simulink model "main"  (R2021a)
settings: Solver=ode45  StartTime=0.0  StopTime=300  RelTol=1e-3
undefined symbols (not defined in the file or in its folder): Discrete, Earth, Time, WGS84
libraries: pid_lib x7, dspvision x5, simulink x2, dspindex x2, ctrlSharedLib x1, aerolibfltsims x1, aerolibtransform2 x1, dspsnks4 x1
(part 1 of 2)
settings Model: SimulationMode=accelerator  Creator=ZumoArthicha  LastModifiedBy=ZumoArthicha

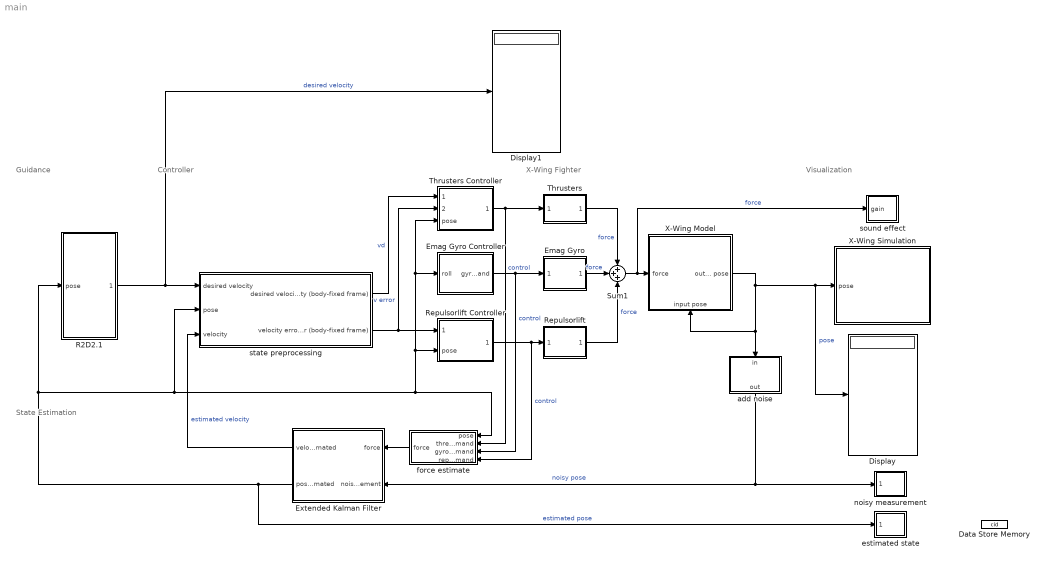
== system main ==
  note: Guidance
  note: Controller
  note: Visualization
  note: X-Wing Fighter
  note: State Estimation
  Data Store Memory : DataStoreMemory  DataStoreName=cid  ReadBeforeWriteMsg=warning  WriteAfterWriteMsg=warning  WriteAfterReadMsg=warning  ShowAdditionalParam=off
  Display : Display
  Display1 : Display
  Emag Gyro : Subsystem
      mask Display: image(imread("pictures/electromagneticgyro.PNG"))
  Emag Gyro Controller : Subsystem
      mask Display: image(imread("pictures/electromagneticgyro.PNG"))
  Extended Kalman Filter : Subsystem
      mask Display: image(imread("pictures/kalman.PNG"))
  R2D2.1 : Subsystem
      mask Display: image(imread("pictures/R2D2_crazy.PNG"))
  Repulsorlift : Subsystem
      mask Display: image(imread("pictures/repulserlift.PNG"))
  Repulsorlift Controller : Subsystem
      mask Display: image(imread("pictures/repulserlift.PNG"))
  Sum1 : Sum  Inputs=+++
  Thrusters : Subsystem
      mask Display: image(imread("pictures/thrusters.PNG"))
  Thrusters Controller : Subsystem
      mask Display: image(imread("pictures/thrusters.PNG"))
  X-Wing Model : Subsystem
      settings: PortSchema="{\"entries\":[{\"content\":{\"sides\":[{\"content\":{\"connectorIds\":[\"In1\"]},\"type\":\"ConnectorPlacement.EquallySpacedRectSide\",\"uuid\":\"9b8fdf7d-c3f6-4599-b802-210579db8a0c\"},{\"content\":{\"connectorIds\":[\"Out1\"],\"side\":\"RIGHT\"},\"type\":\"ConnectorPlacement.EquallySpacedRectSide\",\"uuid\":\"64fce1f1-7921-46e2-bebf-614926f0f3ad\"},{\"content\":{\"connectorIds\":[],\"side\":\"TOP\"},\"type\":\"ConnectorPlacement.EquallySpacedRectSide\",\"uuid\":\"e545f28f-71e6-4ea6-95f8-1eb7e380d19b\"},{\"content\":{\"connectorIds\":[\"In2\"],\"side\":\"BOTTOM\"},\"type\":\"ConnectorPlacement.EquallySpacedRectSide\",\"uuid\":\"bfd9a8ec-cd4d-4e0d-ab0a-253386349908\"}]},\"type\":\"ConnectorPlacement.EquallySpacedConnector\",\"uuid\":\"b40ebf44-1443-4f81-b67e-9daee8e56b53\"}],\"packageUris\":[\"http://schema.mathworks.com/mf0/Connector/R2020b\"],\"version\":\"1.0\"}"
      mask Display: image(imread("pictures/simplified_model.png"))
  X-Wing Simulation : Subsystem
      mask Display: image(imread("pictures/simulation.PNG"))
  add noise : Subsystem
      settings: PortSchema="{\"entries\":[{\"content\":{\"sides\":[{\"content\":{\"connectorIds\":[]},\"type\":\"ConnectorPlacement.EquallySpacedRectSide\",\"uuid\":\"f30e32c1-a276-4dc3-be84-096135bc4245\"},{\"content\":{\"connectorIds\":[],\"side\":\"RIGHT\"},\"type\":\"ConnectorPlacement.EquallySpacedRectSide\",\"uuid\":\"4791b214-a858-4f7a-9932-cf1e7f19f03d\"},{\"content\":{\"connectorIds\":[\"In1\"],\"side\":\"TOP\"},\"type\":\"ConnectorPlacement.EquallySpacedRectSide\",\"uuid\":\"5d6a58a2-1496-42ba-b7c9-fa854909925b\"},{\"content\":{\"connectorIds\":[\"Out1\"],\"side\":\"BOTTOM\"},\"type\":\"ConnectorPlacement.EquallySpacedRectSide\",\"uuid\":\"4cc45cbe-4744-429a-bad1-818b1ea51f93\"}]},\"type\":\"ConnectorPlacement.EquallySpacedConnector\",\"uuid\":\"9c6af004-83db-43a3-a1c2-cc96f6fd9fdc\"}],\"packageUris\":[\"http://schema.mathworks.com/mf0/Connector/R2020b\"],\"version\":\"1.0\"}"
      mask Display: image(imread("pictures/force.jpg"))
  estimated state : Subsystem
      mask Display: image(imread("pictures/xy_graph.png"))
  force estimate : Subsystem
      mask Display: image('D:\SDU\courses\F22_GuidanceNavigationAndControl\project\workspace\pictures\computer.jpg'); % Use "Edit Image" on toolstrip to change.
  noisy measurement : Subsystem
      mask Display: image(imread("pictures/xy_graph.png"))
  sound effect : Subsystem
      mask Display: image(imread("pictures/audio.PNG"))
  state preprocessing : Subsystem
  wires:
  X-Wing Model/1(output pose) -> X-Wing Model/2(input pose), add noise/1(in), Display/1, X-Wing Simulation/1(pose)  "pose"
  Thrusters Controller/1(thrusters command) -> Thrusters/1(threster command), force estimate/2(threster command)  "control"
  Repulsorlift Controller/1(repulsorlift command) -> force estimate/4(repulsorlift command), Repulsorlift/1(repulsorlift command)  "control"
  state preprocessing/1(desired velocity (body-fixed frame)) -> Thrusters Controller/1(desired velocity)  "vd"
  R2D2.1/1(desired velocity) -> Display1/1, state preprocessing/1(desired velocity)  "desired velocity"
  Emag Gyro Controller/1(gyros command) -> force estimate/3(gyros command), Emag Gyro/1(gyros command)  "control"
  Sum1/1 -> sound effect/1(gain), X-Wing Model/1(force)  "force"
  add noise/1(out) -> Extended Kalman Filter/2(noisy measurement), noisy measurement/1(" ")  "noisy pose"
  Extended Kalman Filter/2(pose estimated) -> R2D2.1/1(pose), state preprocessing/2(pose), force estimate/1(pose), Repulsorlift Controller/2(pose), Emag Gyro Controller/1(roll), Thrusters Controller/3(pose), estimated state/1(" ")  "estimated pose"
  Extended Kalman Filter/1(velocity estimated) -> state preprocessing/3(velocity)  "estimated velocity"
  Repulsorlift/1(repulsorlift force) -> Sum1/3  "force"
  Emag Gyro/1(gyros force) -> Sum1/2  "force"
  Thrusters/1(combined thrusters force) -> Sum1/1  "force"
  force estimate/1(force) -> Extended Kalman Filter/1(force)
  state preprocessing/2(velocity error (body-fixed frame)) -> Thrusters Controller/2(velocity error (body-fixed frame)), Repulsorlift Controller/1(vz error)  "v error"

== system main/Emag Gyro ==
  gyros command : Inport
  gyros force : Outport  PortDimensions=6
  wires:
  gyros command/1 -> gyros force/1

== system main/Emag Gyro Controller ==
  roll : Inport
  Constant : Constant  Value=0
  Demux5 : Demux  Outputs=6
  Gain : Gain  Gain=1e4
  Gyros PID : pid_lib/PID Controller  Controller=PID  Form=Parallel  TimeDomain=Continuous-time  UseExternalTs=off  SampleTime=-1  IntegratorMethod=Forward Euler  FilterMethod=Forward Euler  ControllerParametersSource=internal  P=0.5  I=0  D=1  UseFilter=on  N=100  TunerSelectOption=Transfer Function Based (PID Tuner App)  InitialConditionSource=internal  InitialConditionForIntegrator=0  InitialConditionForFilter=0  DifferentiatorICPrevScaledInput=0  ExternalReset=none  TrackingMode=off  Kt=1  LimitOutput=off  SatLimitsSource=internal  UpperSaturationLimit=inf  LowerSaturationLimit=-inf  LinearizeAsGain=on  AntiWindupMode=none  Kb=1  POutMin=[]  POutMax=[]  IOutMin=[]  IOutMax=[]  DOutMin=[]  DOutMax=[]  NOutMin=[]  NOutMax=[]  SumOutMin=[]  SumOutMax=[]  SaturationOutMin=[]  SaturationOutMax=[]  PParamMin=[]  PParamMax=[]  IParamMin=[]  IParamMax=[]  DParamMin=[]  DParamMax=[]  NParamMin=[]  NParamMax=[]  KbParamMin=[]  KbParamMax=[]  KtParamMin=[]  KtParamMax=[]  KbOutMin=[]  KbOutMax=[]  KtOutMin=[]  KtOutMax=[]  IntegratorOutMin=[]  IntegratorOutMax=[]  FilterOutMin=[]  FilterOutMax=[]  SumI1OutMin=[]  SumI1OutMax=[]  SumI2OutMin=[]  SumI2OutMax=[]  SumI3OutMin=[]  SumI3OutMax=[]  SumI4OutMin=[]  SumI4OutMax=[]  SumDOutMin=[]  SumDOutMax=[]  DifferentiatorOutMin=[]  DifferentiatorOutMax=[]  FilterDiffOutCoefMin=[]  FilterDiffOutCoefMax=[]  ReciprocalOutMin=[]  ReciprocalOutMax=[]  SumDenOutMin=[]  SumDenOutMax=[]  SumNumOutMin=[]  SumNumOutMax=[]  DivideOutMin=[]  DivideOutMax=[]  UdiffTsProdOutMin=[]  UdiffTsProdOutMax=[]  NTsProdOutMin=[]  NTsProdOutMax=[]  UintegralTsProdOutMin=[]  UintegralTsProdOutMax=[]  UngainTsProdOutMin=[]  UngainTsProdOutMax=[]  IntegratorContinuousStateAttributes=''  IntegratorStateMustResolveToSignalObject=off  IntegratorRTWStateStorageClass=Auto  FilterContinuousStateAttributes=''  FilterStateMustResolveToSignalObject=off  FilterRTWStateStorageClass=Auto  ParallelPVariant=InternalParameters  IdealPVariant=Disabled  IVariant=InternalParameters  DVariant=InternalParameters  IntegratorVariant=Continuous  SatVariant=Disabled  AWVariant=Passthrough  PCopyVariant=Disabled  TRVariant=Disabled  FdbkBlocksVariant=Forward  IdealPFdbkVariant=Disabled  SatFdbkVariant=Disabled  DerivativeFilterVariant=ContFilter  NVariant=InternalParameters  NCopyVariant=Disabled  FilterICVariant=InternalICsFilter  IntegratorICVariant=InternalICs  ExternalResetVariant=Disabled  TRSumVariant=Passthrough  SumFdbkVariant=Disabled  SumVariant=Sum_PID  TsampFilterVariant=InternalTs  TsampNgainVariant=Passthrough  TsampIntegralVariant=Passthrough  ExternalSaturationOutDataTypeStr=Inherit: Same as second input
  Product : Product
  Sum : Sum  Inputs=|+-
  directional constrain : Constant  Value=[0;0;0;1;0;0]  VectorParams1D=off
  gyros command : Outport  PortDimensions=6
  wires:
  directional constrain/1 -> Product/1  "directional constrain"
  Gain/1 -> Product/2
  Sum/1 -> Gyros PID/1  "roll error"
  Constant/1 -> Sum/1
  roll/1 -> Demux5/1
  Demux5/4 -> Sum/2
  Gyros PID/1 -> Gain/1
  Product/1 -> gyros command/1

== system main/Extended Kalman Filter ==
  force : Inport
  noisy measurement : Inport  Port=2
  Kalman Filter : Subsystem
      mask Display: image(imread("pictures/kalman.PNG"))
  To File : ToFile  Filename=pose.mat  MatrixName=data  SaveFormat=Timeseries
  input linearization : Subsystem
      mask Display: image(imread("pictures/equations/linearization.PNG"))
  velocity estimated : Outport
  pose estimated : Outport  Port=2
  wires:
  input linearization/1(force1) -> Kalman Filter/1(force)
  Kalman Filter/2(estimated velocity) -> velocity estimated/1  "velocity estimated"
  Kalman Filter/1(estimated pose) -> To File/1, input linearization/1(pose), pose estimated/1  "pose estimated"
  force/1 -> input linearization/2(force)
  noisy measurement/1 -> Kalman Filter/2(measure)

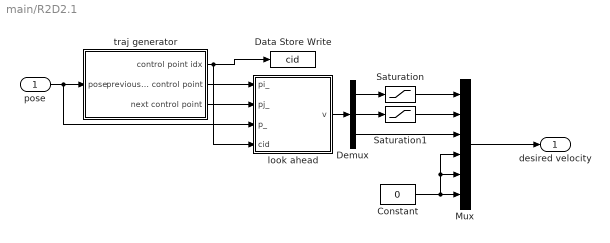
== system main/R2D2.1 ==
  pose : Inport
  Constant : Constant  Value=0
  Data Store Write : DataStoreWrite  DataStoreName=cid  IndexOptions=Index vector (dialog)  Indices=1  OutputSizes=1
  Demux : Demux  Outputs=3
  Mux : Mux  Inputs=6
  Saturation : Saturate  UpperLimit=100  LowerLimit=-100
  Saturation1 : Saturate  UpperLimit=100  LowerLimit=-100
  look ahead : MATLAB Function  TreatAsAtomicUnit=on
  traj generator : Subsystem
  desired velocity : Outport
  wires:
  traj generator/3(next control point) -> look ahead/2(pj_)
  pose/1 -> look ahead/3(p_), traj generator/1(pose)
  traj generator/2(previous control point) -> look ahead/1(pi_)
  look ahead/1(v) -> Demux/1
  Demux/3 -> Mux/3
  Constant/1 -> Mux/4, Mux/5, Mux/6
  Mux/1 -> desired velocity/1
  traj generator/1(control point idx) -> Data Store Write/1, look ahead/4(cid)
  Demux/2 -> Saturation1/1
  Demux/1 -> Saturation/1
  Saturation/1 -> Mux/1
  Saturation1/1 -> Mux/2

== system main/Repulsorlift ==
  repulsorlift command : Inport
  repulsorlift force : Outport  PortDimensions=6
  wires:
  repulsorlift command/1 -> repulsorlift force/1

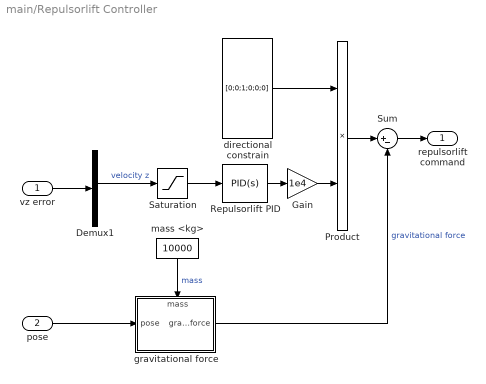
== system main/Repulsorlift Controller ==
  vz error : Inport
  pose : Inport  Port=2
  Demux1 : Demux  Outputs=6
  Gain : Gain  Gain=1e4
  Product : Product
  Repulsorlift PID : pid_lib/PID Controller  Controller=PID  Form=Parallel  TimeDomain=Continuous-time  UseExternalTs=off  SampleTime=-1  IntegratorMethod=Forward Euler  FilterMethod=Forward Euler  ControllerParametersSource=internal  P=0.01  I=0  D=0.1  UseFilter=on  N=100  TunerSelectOption=Transfer Function Based (PID Tuner App)  InitialConditionSource=internal  InitialConditionForIntegrator=0  InitialConditionForFilter=0  DifferentiatorICPrevScaledInput=0  ExternalReset=none  TrackingMode=off  Kt=1  LimitOutput=off  SatLimitsSource=internal  UpperSaturationLimit=inf  LowerSaturationLimit=-inf  LinearizeAsGain=on  AntiWindupMode=none  Kb=1  POutMin=[]  POutMax=[]  IOutMin=[]  IOutMax=[]  DOutMin=[]  DOutMax=[]  NOutMin=[]  NOutMax=[]  SumOutMin=[]  SumOutMax=[]  SaturationOutMin=[]  SaturationOutMax=[]  PParamMin=[]  PParamMax=[]  IParamMin=[]  IParamMax=[]  DParamMin=[]  DParamMax=[]  NParamMin=[]  NParamMax=[]  KbParamMin=[]  KbParamMax=[]  KtParamMin=[]  KtParamMax=[]  KbOutMin=[]  KbOutMax=[]  KtOutMin=[]  KtOutMax=[]  IntegratorOutMin=[]  IntegratorOutMax=[]  FilterOutMin=[]  FilterOutMax=[]  SumI1OutMin=[]  SumI1OutMax=[]  SumI2OutMin=[]  SumI2OutMax=[]  SumI3OutMin=[]  SumI3OutMax=[]  SumI4OutMin=[]  SumI4OutMax=[]  SumDOutMin=[]  SumDOutMax=[]  DifferentiatorOutMin=[]  DifferentiatorOutMax=[]  FilterDiffOutCoefMin=[]  FilterDiffOutCoefMax=[]  ReciprocalOutMin=[]  ReciprocalOutMax=[]  SumDenOutMin=[]  SumDenOutMax=[]  SumNumOutMin=[]  SumNumOutMax=[]  DivideOutMin=[]  DivideOutMax=[]  UdiffTsProdOutMin=[]  UdiffTsProdOutMax=[]  NTsProdOutMin=[]  NTsProdOutMax=[]  UintegralTsProdOutMin=[]  UintegralTsProdOutMax=[]  UngainTsProdOutMin=[]  UngainTsProdOutMax=[]  IntegratorContinuousStateAttributes=''  IntegratorStateMustResolveToSignalObject=off  IntegratorRTWStateStorageClass=Auto  FilterContinuousStateAttributes=''  FilterStateMustResolveToSignalObject=off  FilterRTWStateStorageClass=Auto  ParallelPVariant=InternalParameters  IdealPVariant=Disabled  IVariant=InternalParameters  DVariant=InternalParameters  IntegratorVariant=Continuous  SatVariant=Disabled  AWVariant=Passthrough  PCopyVariant=Disabled  TRVariant=Disabled  FdbkBlocksVariant=Forward  IdealPFdbkVariant=Disabled  SatFdbkVariant=Disabled  DerivativeFilterVariant=ContFilter  NVariant=InternalParameters  NCopyVariant=Disabled  FilterICVariant=InternalICsFilter  IntegratorICVariant=InternalICs  ExternalResetVariant=Disabled  TRSumVariant=Passthrough  SumFdbkVariant=Disabled  SumVariant=Sum_PID  TsampFilterVariant=InternalTs  TsampNgainVariant=Passthrough  TsampIntegralVariant=Passthrough  ExternalSaturationOutDataTypeStr=Inherit: Same as second input
  Saturation : Saturate  UpperLimit=10  LowerLimit=-10
  Sum : Sum  Inputs=|+-
  directional constrain : Constant  Value=[0;0;1;0;0;0]  VectorParams1D=off
  gravitational force : Subsystem
      settings: PortSchema="{\"entries\":[{\"content\":{\"sides\":[{\"content\":{\"connectorIds\":[\"In1\"]},\"type\":\"ConnectorPlacement.EquallySpacedRectSide\",\"uuid\":\"d93db66b-fcc6-4c17-9134-40d9beba2643\"},{\"content\":{\"connectorIds\":[\"Out1\"],\"side\":\"RIGHT\"},\"type\":\"ConnectorPlacement.EquallySpacedRectSide\",\"uuid\":\"70571ecc-e0da-42b3-8b7b-d4ce677f32d8\"},{\"content\":{\"connectorIds\":[\"In2\"],\"side\":\"TOP\"},\"type\":\"ConnectorPlacement.EquallySpacedRectSide\",\"uuid\":\"56b2d7be-0ac4-47dc-afb8-3ce057fd0ced\"},{\"content\":{\"connectorIds\":[],\"side\":\"BOTTOM\"},\"type\":\"ConnectorPlacement.EquallySpacedRectSide\",\"uuid\":\"175b75d5-a12f-4632-9256-2a0db7457e72\"}]},\"type\":\"ConnectorPlacement.EquallySpacedConnector\",\"uuid\":\"6f54763d-dba9-4fd6-aa24-fb7b6af2d4a1\"}],\"packageUris\":[\"http://schema.mathworks.com/mf0/Connector/R2020b\"],\"version\":\"1.0\"}"
      mask Display: image(imread("pictures/gravitational_force.PNG"))
  mass <kg> : Constant  Value=10000
  repulsorlift command : Outport  PortDimensions=6
  wires:
  directional constrain/1 -> Product/1
  Repulsorlift PID/1 -> Gain/1
  Product/1 -> Sum/1
  Sum/1 -> repulsorlift command/1
  Gain/1 -> Product/2
  Saturation/1 -> Repulsorlift PID/1
  vz error/1 -> Demux1/1
  Demux1/3 -> Saturation/1  "velocity z"
  mass <kg>/1 -> gravitational force/2(mass)  "mass"
  pose/1 -> gravitational force/1(pose)
  gravitational force/1(gravitational force) -> Sum/2  "gravitational force"

== system main/Thrusters ==
  threster command : Inport  PortDimensions=4
  Matrix Multiply2 : Product  Multiplication=Matrix(*)
  thrust matrix : Constant  Value=[0.25 0.25 0.25 0.25; 0 0 0 0; 0 0 0 0; 0 0 0 0; -0.68 -0.68 0.68 0.68; 1.425 -1.425 1.425 -1.425]  VectorParams1D=off
  combined thrusters force : Outport  PortDimensions=6
  wires:
  thrust matrix/1 -> Matrix Multiply2/1
  Matrix Multiply2/1 -> combined thrusters force/1  "low-level thruster command"
  threster command/1 -> Matrix Multiply2/2

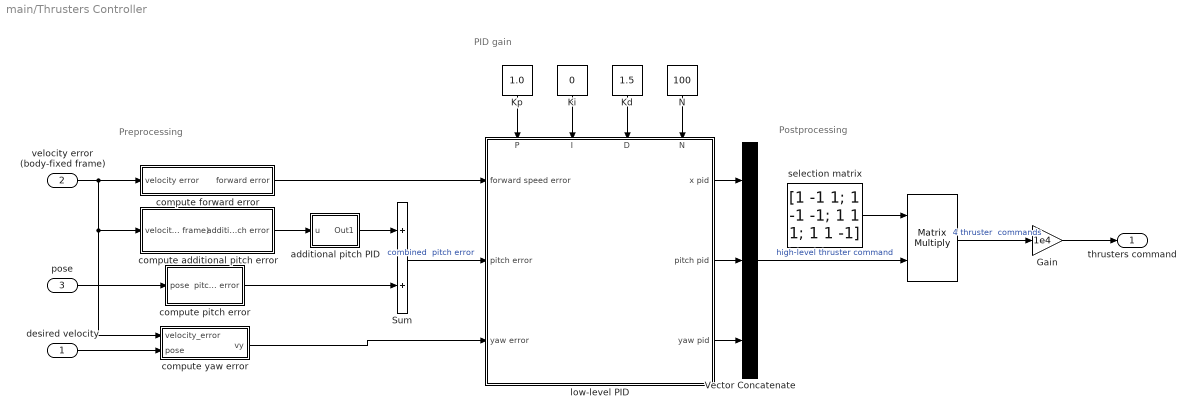
== system main/Thrusters Controller ==
  note: Postprocessing
  note: Preprocessing
  note: PID gain
  desired velocity : Inport
  velocity error (body-fixed frame) : Inport  Port=2
  pose : Inport  Port=3
  "  " : Product  Multiplication=Matrix(*)
  Gain : Gain  Gain=1e4
  Kd : Constant  Value=1.5
  Ki : Constant  Value=0
  Kp : Constant  Value=1.0
  N : Constant  Value=100
  Sum : Sum
  Vector Concatenate : Concatenate  NumInputs=3
  additional pitch PID : Subsystem
  compute additional pitch error : Subsystem
  compute forward error : Subsystem
  compute pitch error : Subsystem
  compute yaw error : Subsystem
  low-level PID : Subsystem
      settings: PortSchema="{\"entries\":[{\"content\":{\"sides\":[{\"content\":{\"connectorIds\":[\"In1\",\"In2\",\"In3\"]},\"type\":\"ConnectorPlacement.EquallySpacedRectSide\",\"uuid\":\"f6ea6f6d-4efd-425d-8a85-ce3b9bde565c\"},{\"content\":{\"connectorIds\":[\"Out1\",\"Out2\",\"Out3\"],\"side\":\"RIGHT\"},\"type\":\"ConnectorPlacement.EquallySpacedRectSide\",\"uuid\":\"bea2efba-fcca-41fe-8e46-9fa204d644b4\"},{\"content\":{\"connectorIds\":[\"In4\",\"In5\",\"In6\",\"In7\"],\"side\":\"TOP\"},\"type\":\"ConnectorPlacement.EquallySpacedRectSide\",\"uuid\":\"c7db24d1-2300-4d89-a06d-38d8ccf635f0\"}]},\"type\":\"ConnectorPlacement.EquallySpacedConnector\",\"uuid\":\"54c313d2-af5a-49ea-a2f4-4d36f80b668a\"}],\"packageUris\":[\"http://schema.mathworks.com/mf0/Connector/R2020b\"],\"version\":\"1.0\"}"
  selection matrix : Constant  Value=[1 -1 1; 1 -1 -1; 1 1 1; 1 1 -1]  VectorParams1D=off
  thrusters command : Outport  PortDimensions=4
  wires:
  Kp/1 -> low-level PID/4(P)
  selection matrix/1 -> "  "/1
  Vector Concatenate/1 -> "  "/2  "high-level thruster command"
  pose/1 -> compute pitch error/1(pose)
  compute pitch error/1(pitch error) -> Sum/2
  velocity error (body-fixed frame)/1 -> compute yaw error/1(velocity_error), compute additional pitch error/1(velocity error (world-fixed frame)), compute forward error/1(velocity error)
  desired velocity/1 -> compute yaw error/2(pose)
  compute additional pitch error/1(addition pitch error) -> additional pitch PID/1(u)
  additional pitch PID/1(Out1) -> Sum/1
  Ki/1 -> low-level PID/5(I)
  Kd/1 -> low-level PID/6(D)
  N/1 -> low-level PID/7(N)
  compute forward error/1(forward error) -> low-level PID/1(forward speed error)
  Sum/1 -> low-level PID/2(pitch error)  "combined  pitch error"
  compute yaw error/1(vy) -> low-level PID/3(yaw error)
  low-level PID/1(x pid) -> Vector Concatenate/1
  low-level PID/2(pitch pid) -> Vector Concatenate/2
  low-level PID/3(yaw pid) -> Vector Concatenate/3
  "  "/1 -> Gain/1  "4 thruster  commands"
  Gain/1 -> thrusters command/1

== system main/X-Wing Model ==
  force : Inport
  input pose : Inport  Port=2
  Sum : Sum  Inputs=++|
  X-wing Model : Subsystem
      settings: PortSchema="{\"entries\":[{\"content\":{\"sides\":[{\"content\":{\"connectorIds\":[\"In1\"]},\"type\":\"ConnectorPlacement.EquallySpacedRectSide\",\"uuid\":\"7004d7e2-eb30-41ed-9d5e-f00159415fc4\"},{\"content\":{\"connectorIds\":[\"Out1\",\"Out2\"],\"side\":\"RIGHT\"},\"type\":\"ConnectorPlacement.EquallySpacedRectSide\",\"uuid\":\"4cf7ba01-0c86-439c-9faf-473746ab50fc\"},{\"content\":{\"connectorIds\":[\"In2\",\"In3\"],\"side\":\"TOP\"},\"type\":\"ConnectorPlacement.EquallySpacedRectSide\",\"uuid\":\"4a15a873-16d7-4740-9282-1fecb26c48e4\"},{\"content\":{\"connectorIds\":[],\"side\":\"BOTTOM\"},\"type\":\"ConnectorPlacement.EquallySpacedRectSide\",\"uuid\":\"87e73f3e-eb46-42cc-8158-d40318a5aa75\"}]},\"type\":\"ConnectorPlacement.EquallySpacedConnector\",\"uuid\":\"64dad74e-3dd4-4677-9bab-84aaaaaa8f26\"}],\"packageUris\":[\"http://schema.mathworks.com/mf0/Connector/R2020b\"],\"version\":\"1.0\"}"
      mask Display: image(imread("pictures/simplified_model.png"))
  gravitational force : Subsystem
      settings: PortSchema="{\"entries\":[{\"content\":{\"sides\":[{\"content\":{\"connectorIds\":[\"In1\"]},\"type\":\"ConnectorPlacement.EquallySpacedRectSide\",\"uuid\":\"d93db66b-fcc6-4c17-9134-40d9beba2643\"},{\"content\":{\"connectorIds\":[\"Out1\"],\"side\":\"RIGHT\"},\"type\":\"ConnectorPlacement.EquallySpacedRectSide\",\"uuid\":\"70571ecc-e0da-42b3-8b7b-d4ce677f32d8\"},{\"content\":{\"connectorIds\":[\"In2\"],\"side\":\"TOP\"},\"type\":\"ConnectorPlacement.EquallySpacedRectSide\",\"uuid\":\"56b2d7be-0ac4-47dc-afb8-3ce057fd0ced\"},{\"content\":{\"connectorIds\":[],\"side\":\"BOTTOM\"},\"type\":\"ConnectorPlacement.EquallySpacedRectSide\",\"uuid\":\"175b75d5-a12f-4632-9256-2a0db7457e72\"}]},\"type\":\"ConnectorPlacement.EquallySpacedConnector\",\"uuid\":\"6f54763d-dba9-4fd6-aa24-fb7b6af2d4a1\"}],\"packageUris\":[\"http://schema.mathworks.com/mf0/Connector/R2020b\"],\"version\":\"1.0\"}"
      mask Display: image(imread("pictures/gravitational_force.PNG"))
  innertia <kg m2> : Constant  Value=[36145 0 0; 2.26927 116437.915354 0.00035374516; 0 0.00035374516 90590.2796914]  VectorParams1D=off
  mass <kg> : Constant  Value=10000
  output pose : Outport
  wires:
  mass <kg>/1 -> gravitational force/2(mass), X-wing Model/2(mass)  "mass"
  innertia <kg m2>/1 -> X-wing Model/3(inertia)  "inertia"
  X-wing Model/1(pose) -> output pose/1  "pose"
  input pose/1 -> gravitational force/1(pose)  "pose"
  Sum/1 -> X-wing Model/1(force)  "force"
  force/1 -> Sum/1
  gravitational force/1(gravitational force) -> Sum/2  "gravitational force"

== system main/X-Wing Simulation ==
  pose : Inport
  Constant1 : Constant  Value=[30;300;100]  VectorParams1D=off
  Demux : Demux  Outputs=2
  FlightGear Simulation : aerolibfltsims/FlightGear Preconfigured 6DoF Animation  xFlightGearVersion=v2019.1  DestinationIpAddress=127.0.0.1  DestinationPort=5502  SampleTime=1/20  packetVersion=24  mask(FlightGearQuick6DoFAnimation){}
      mask Display:
      | % This is a new mask on top of the base mask.
      | % Use "View base mask" link below to see the base mask.
      | image(imread("pictures/simulation.PNG"))
  MATLAB Function : MATLAB Function  TreatAsAtomicUnit=on
  Mux1 : Mux  Inputs=2
  flat earth 2 LLA : Subsystem
  special : Subsystem
  wires:
  MATLAB Function/1(pose_) -> FlightGear Simulation/1
  pose/1 -> Demux/1
  Demux/2 -> Mux1/2
  Mux1/1 -> MATLAB Function/1(pose)
  Constant1/1 -> flat earth 2 LLA/1(multiplication gain)
  Demux/1 -> flat earth 2 LLA/2(position (flat))
  flat earth 2 LLA/1(position (LLA)) -> Mux1/1

== system main/add noise ==
  in : Inport
  Measurement Noise : Subsystem
  Sum : Sum  Inputs=|++
  To File1 : ToFile  Filename=noisypose.mat  MatrixName=data  SaveFormat=Timeseries
  To File3 : ToFile  Filename=truepose.mat  MatrixName=data  SaveFormat=Timeseries
  out : Outport
  wires:
  Measurement Noise/1(nois) -> Sum/2
  in/1 -> To File3/1, Sum/1
  Sum/1 -> To File1/1, out/1  "measurement"

== system main/estimated state ==
  " " : Inport
  Demux3 : Demux  Outputs=6
  XY Graph : simulink/Sinks/XY Graph  xmin=-0.2  xmax=1  ymin=-0.2  ymax=1  st=-1
  scaling gain : Gain  Gain=2e-4
  wires:
  Demux3/1 -> XY Graph/1  "x"
  Demux3/2 -> XY Graph/2  "y"
  scaling gain/1 -> Demux3/1
  " "/1 -> scaling gain/1

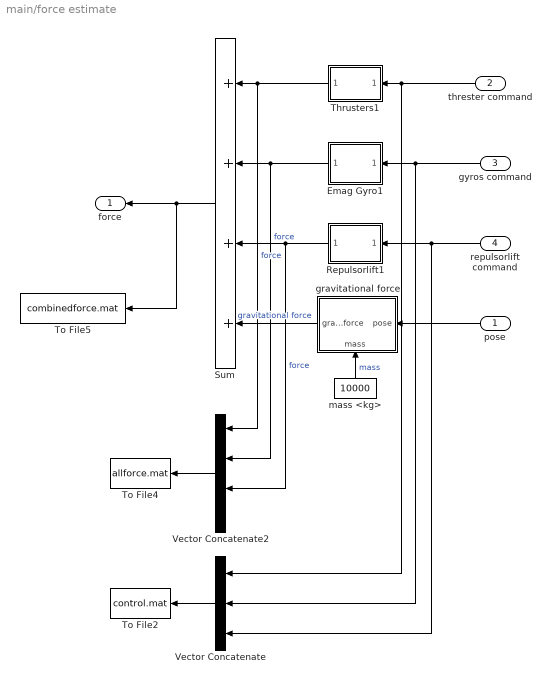
== system main/force estimate ==
  pose : Inport
  threster command : Inport  Port=2
  gyros command : Inport  Port=3
  repulsorlift command : Inport  Port=4
  Emag Gyro1 : Subsystem
      mask Display: image(imread("pictures/electromagneticgyro.PNG"))
  Repulsorlift1 : Subsystem
      mask Display: image(imread("pictures/repulserlift.PNG"))
  Sum : Sum  Inputs=++++
  Thrusters1 : Subsystem
      mask Display: image(imread("pictures/thrusters.PNG"))
  To File2 : ToFile  Filename=control.mat  MatrixName=data  SaveFormat=Timeseries
  To File4 : ToFile  Filename=allforce.mat  MatrixName=data  SaveFormat=Timeseries
  To File5 : ToFile  Filename=combinedforce.mat  MatrixName=data  SaveFormat=Timeseries
  Vector Concatenate : Concatenate  NumInputs=3
  Vector Concatenate2 : Concatenate  NumInputs=4
  gravitational force : Subsystem
      settings: PortSchema="{\"entries\":[{\"content\":{\"sides\":[{\"content\":{\"connectorIds\":[\"In1\"]},\"type\":\"ConnectorPlacement.EquallySpacedRectSide\",\"uuid\":\"d93db66b-fcc6-4c17-9134-40d9beba2643\"},{\"content\":{\"connectorIds\":[\"Out1\"],\"side\":\"RIGHT\"},\"type\":\"ConnectorPlacement.EquallySpacedRectSide\",\"uuid\":\"70571ecc-e0da-42b3-8b7b-d4ce677f32d8\"},{\"content\":{\"connectorIds\":[],\"side\":\"TOP\"},\"type\":\"ConnectorPlacement.EquallySpacedRectSide\",\"uuid\":\"56b2d7be-0ac4-47dc-afb8-3ce057fd0ced\"},{\"content\":{\"connectorIds\":[\"In2\"],\"side\":\"BOTTOM\"},\"type\":\"ConnectorPlacement.EquallySpacedRectSide\",\"uuid\":\"175b75d5-a12f-4632-9256-2a0db7457e72\"}]},\"type\":\"ConnectorPlacement.EquallySpacedConnector\",\"uuid\":\"6f54763d-dba9-4fd6-aa24-fb7b6af2d4a1\"}],\"packageUris\":[\"http://schema.mathworks.com/mf0/Connector/R2020b\"],\"version\":\"1.0\"}"
      mask Display: image(imread("pictures/gravitational_force.PNG"))
  mass <kg> : Constant  Value=10000
  force : Outport
  wires:
  gyros command/1 -> Vector Concatenate/2, Emag Gyro1/1(gyros command)
  threster command/1 -> Vector Concatenate/1, Thrusters1/1(threster command)
  repulsorlift command/1 -> Vector Concatenate/3, Repulsorlift1/1(repulsorlift command)
  Sum/1 -> To File5/1, force/1
  Emag Gyro1/1(gyros force) -> Vector Concatenate2/2, Sum/2  "force"
  Thrusters1/1(combined thrusters force) -> Vector Concatenate2/1, Sum/1  "force"
  Repulsorlift1/1(repulsorlift force) -> Vector Concatenate2/3, Sum/3  "force"
  Vector Concatenate2/1 -> To File4/1
  Vector Concatenate/1 -> To File2/1
  gravitational force/1(gravitational force) -> Sum/4  "gravitational force"
  pose/1 -> gravitational force/1(pose)
  mass <kg>/1 -> gravitational force/2(mass)  "mass"

== system main/noisy measurement ==
  " " : Inport
  Demux3 : Demux  Outputs=6
  XY Graph : simulink/Sinks/XY Graph  xmin=-0.2  xmax=1  ymin=-0.2  ymax=1  st=-1
  scaling gain : Gain  Gain=2e-4
  wires:
  Demux3/1 -> XY Graph/1  "x"
  Demux3/2 -> XY Graph/2  "y"
  scaling gain/1 -> Demux3/1
  " "/1 -> scaling gain/1

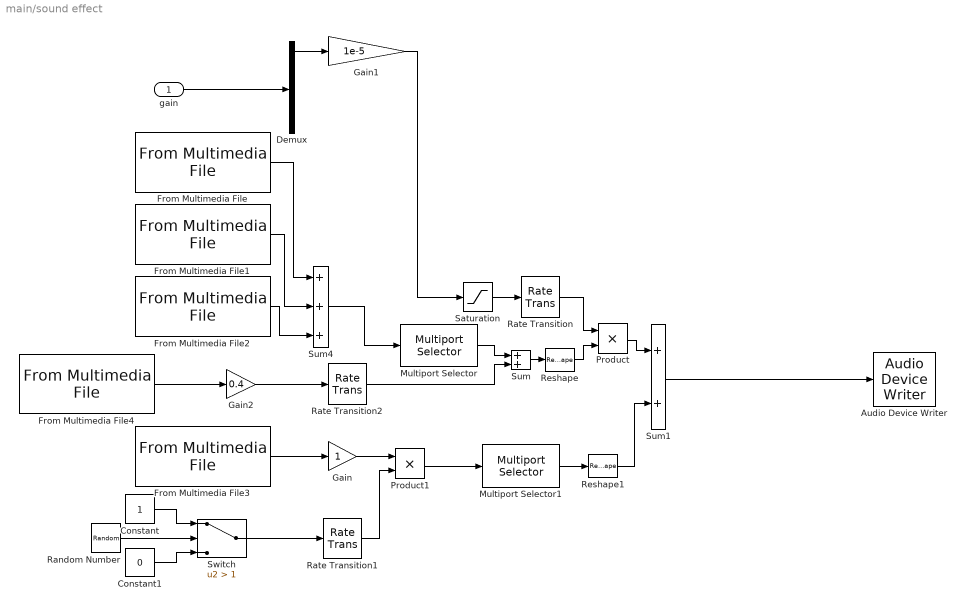
== system main/sound effect ==
  gain : Inport
  Audio Device Writer : dspsnks4/Audio Device Writer  Driver=DirectSound  Device=Default  InheritSampleRate=on  SampleRate=44100  BitDepth=16-bit integer  BufferSize=4096  NumBuffers=10  DefaultOutputChannelMapping=on  OutputChannelMapping=1:2  OutputNumUnderrunSamples=off  DriverIdx=1  DeviceWarnFlag=''
  Constant : Constant
  Constant1 : Constant  Value=0
  Demux : Demux  Outputs=6
  From Multimedia File : dspvision/From Multimedia File  inputFilename=D:\SDU\courses\F22_GuidanceNavigationAndControl\project\workspace\sound\XWing-Fly1.wav  readRange=[1 Inf]  loop=on  numPlays=inf  outputStreams=Audio only  videoDataType=single  audioDataType=double  inheritSampleTime=on  userDefinedSampleTime=1/30  noAudioOutput=off  isIntensityVideo=off  fourcc=RGB  colorVideoFormat=One multidimensional signal  outputEOF=off  dataOrg=Column-major  audioFrameSize=1024  computeAudioFrameSize=off  outSamplingMode=Sample based
  From Multimedia File1 : dspvision/From Multimedia File  inputFilename=D:\SDU\courses\F22_GuidanceNavigationAndControl\project\workspace\sound\XWing-Fly2.wav  readRange=[1 Inf]  loop=on  numPlays=inf  outputStreams=Audio only  videoDataType=single  audioDataType=double  inheritSampleTime=on  userDefinedSampleTime=1/30  noAudioOutput=off  isIntensityVideo=off  fourcc=RGB  colorVideoFormat=One multidimensional signal  outputEOF=off  dataOrg=Column-major  audioFrameSize=1024  computeAudioFrameSize=off  outSamplingMode=Sample based
  From Multimedia File2 : dspvision/From Multimedia File  inputFilename=D:\SDU\courses\F22_GuidanceNavigationAndControl\project\workspace\sound\XWing-Fly3.wav  readRange=[1 Inf]  loop=on  numPlays=inf  outputStreams=Audio only  videoDataType=single  audioDataType=double  inheritSampleTime=on  userDefinedSampleTime=1/30  noAudioOutput=off  isIntensityVideo=off  fourcc=RGB  colorVideoFormat=One multidimensional signal  outputEOF=off  dataOrg=Column-major  audioFrameSize=1024  computeAudioFrameSize=off  outSamplingMode=Sample based
  From Multimedia File3 : dspvision/From Multimedia File  inputFilename=D:\SDU\courses\F22_GuidanceNavigationAndControl\project\workspace\sound\XWing-Laser.wav  readRange=[1 Inf]  loop=on  numPlays=inf  outputStreams=Audio only  videoDataType=single  audioDataType=double  inheritSampleTime=on  userDefinedSampleTime=1/30  noAudioOutput=off  isIntensityVideo=off  fourcc=RGB  colorVideoFormat=One multidimensional signal  outputEOF=off  dataOrg=Column-major  audioFrameSize=1024  computeAudioFrameSize=off  outSamplingMode=Sample based
  From Multimedia File4 : dspvision/From Multimedia File  inputFilename=D:\SDU\courses\F22_GuidanceNavigationAndControl\project\workspace\sound\R2D2.mp3  readRange=[1 Inf]  loop=on  numPlays=inf  outputStreams=Audio only  videoDataType=single  audioDataType=double  inheritSampleTime=on  userDefinedSampleTime=1/30  noAudioOutput=off  isIntensityVideo=off  fourcc=RGB  colorVideoFormat=One multidimensional signal  outputEOF=off  dataOrg=Column-major  audioFrameSize=1024  computeAudioFrameSize=off  outSamplingMode=Sample based
  Gain : Gain
  Gain1 : Gain  Gain=1e-5
  Gain2 : Gain  Gain=0.4
  Multiport Selector : dspindex/Multiport Selector  rowsOrCols=Columns  idxCellArray=2  idxErrMode=Clip Index
  Multiport Selector1 : dspindex/Multiport Selector  rowsOrCols=Columns  idxCellArray=2  idxErrMode=Clip Index
  Product : Product
  Product1 : Product
  Random Number : RandomNumber  SampleTime=0.4643990929705216
  Rate Transition : RateTransition
  Rate Transition1 : RateTransition
  Rate Transition2 : RateTransition
  Reshape : Reshape
  Reshape1 : Reshape
  Saturation : Saturate  UpperLimit=1  LowerLimit=0.5
  Sum : Sum
  Sum1 : Sum
  Sum4 : Sum  Inputs=+++
  Switch : Switch  Criteria=u2 > Threshold  Threshold=1
  wires:
  From Multimedia File3/1 -> Gain/1
  From Multimedia File/1 -> Sum4/1
  From Multimedia File2/1 -> Sum4/3
  From Multimedia File1/1 -> Sum4/2
  Product/1 -> Sum1/1
  Sum1/1 -> Audio Device Writer/1
  Sum4/1 -> Multiport Selector/1
  Multiport Selector1/1 -> Reshape1/1
  Demux/1 -> Gain1/1
  gain/1 -> Demux/1
  Gain1/1 -> Saturation/1
  Rate Transition/1 -> Product/1
  Reshape1/1 -> Sum1/2
  Saturation/1 -> Rate Transition/1
  Gain/1 -> Product1/1
  Product1/1 -> Multiport Selector1/1
  Rate Transition1/1 -> Product1/2
  Random Number/1 -> Switch/2
  Constant/1 -> Switch/1
  Constant1/1 -> Switch/3
  Switch/1 -> Rate Transition1/1
  From Multimedia File4/1 -> Gain2/1
  Reshape/1 -> Product/2
  Sum/1 -> Reshape/1
  Multiport Selector/1 -> Sum/1
  Rate Transition2/1 -> Sum/2
  Gain2/1 -> Rate Transition2/1

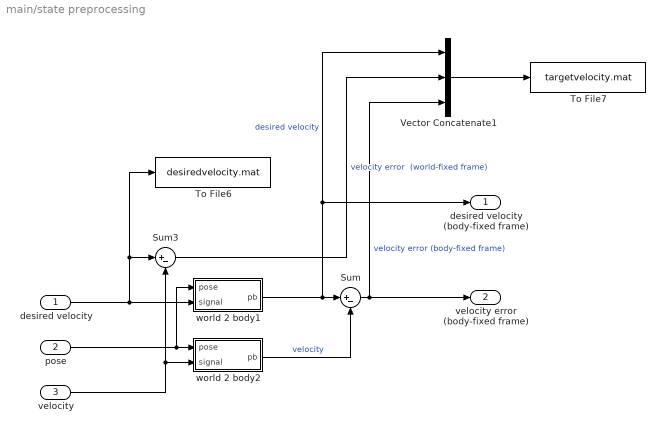
== system main/state preprocessing ==
  desired velocity : Inport
  pose : Inport  Port=2
  velocity : Inport  Port=3
  Sum : Sum  Inputs=|+-
  Sum3 : Sum  Inputs=|+-
  To File6 : ToFile  Filename=desiredvelocity.mat  MatrixName=data  SaveFormat=Timeseries
  To File7 : ToFile  Filename=targetvelocity.mat  MatrixName=data  SaveFormat=Timeseries
  Vector Concatenate1 : Concatenate  NumInputs=3
  world 2 body1 : MATLAB Function  TreatAsAtomicUnit=on
  world 2 body2 : MATLAB Function  TreatAsAtomicUnit=on
  desired velocity (body-fixed frame) : Outport
  velocity error (body-fixed frame) : Outport  Port=2
  wires:
  world 2 body1/1(pb) -> Vector Concatenate1/1, desired velocity (body-fixed frame)/1, Sum/1  "desired velocity"
  desired velocity/1 -> world 2 body1/2(signal), To File6/1, Sum3/1
  Sum/1 -> Vector Concatenate1/3, velocity error (body-fixed frame)/1  "velocity error (body-fixed frame)"
  pose/1 -> world 2 body1/1(pose), world 2 body2/1(pose)
  world 2 body2/1(pb) -> Sum/2  "velocity"
  Sum3/1 -> Vector Concatenate1/2  "velocity error  (world-fixed frame)"
  velocity/1 -> world 2 body2/2(signal), Sum3/2
  Vector Concatenate1/1 -> To File7/1

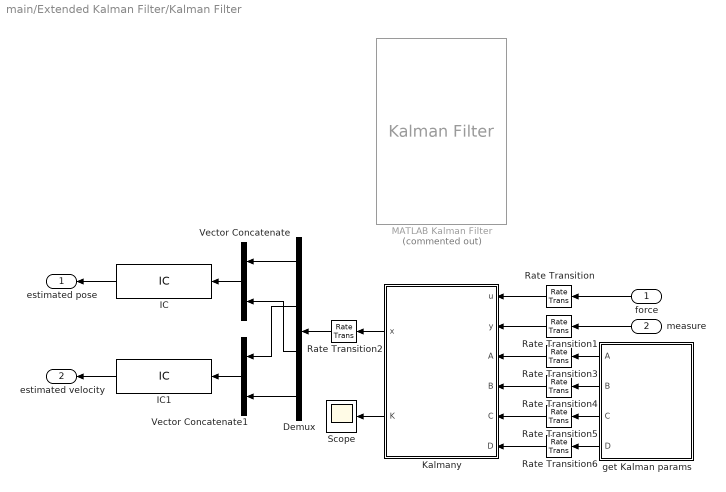
== system main/Extended Kalman Filter/Kalman Filter ==
  force : Inport
  measure : Inport  Port=2
  Demux : Demux
  IC : InitialCondition  Value=[0;0;1.705/100;0;0;0]
  IC1 : InitialCondition  Value=[0;0;0;0;0;0]
  Kalmany : Subsystem
  MATLAB Kalman Filter : ctrlSharedLib/Kalman Filter  Commented=on  TimeDomain=Discrete-Time  UseCurrentEstimator=on  ModelSource=Input port  ModelSourceVariable=ss(0.95,1,1,0,1)  A=0.95  B=1  C=1  D=0  NumberOfStates=12  NumberOfInputs=6  NumberOfOutputs=6  InitialEstimateSource=Dialog  X0=[0;0;1.705/100;0;0;0;0;0;0;0;0;0]  P0=10  UseK=off  UseGH=off  NumberOfProcessNoiseInputs=1  G=1  TimeInvariantG=on  H=0  TimeInvariantH=on  Q=1  TimeInvariantQ=on  R=100  TimeInvariantR=on  N=0  TimeInvariantN=on  AddInputPort=on  AddEnablePort=off  OutputEstimatedY=off  OutputP=off  Ts=0.005
  Rate Transition{,1,3..6} (6 alike) : RateTransition  OutPortSampleTime=0.005
  Rate Transition2 : RateTransition  OutPortSampleTime=0
  Scope : Scope
  Vector Concatenate : Concatenate
  Vector Concatenate1 : Concatenate
  get Kalman params : MATLAB Function  TreatAsAtomicUnit=on
  estimated pose : Outport
  estimated velocity : Outport  Port=2
  wires:
  force/1 -> Rate Transition/1
  measure/1 -> Rate Transition1/1
  Vector Concatenate1/1 -> IC1/1
  Demux/2 -> Vector Concatenate1/1
  Demux/1 -> Vector Concatenate/1
  Demux/3 -> Vector Concatenate/2
  Vector Concatenate/1 -> IC/1
  Demux/4 -> Vector Concatenate1/2
  Rate Transition2/1 -> Demux/1
  IC/1 -> estimated pose/1
  IC1/1 -> estimated velocity/1
  get Kalman params/1(A) -> Rate Transition3/1
  get Kalman params/2(B) -> Rate Transition4/1
  get Kalman params/4(D) -> Rate Transition6/1
  get Kalman params/3(C) -> Rate Transition5/1
  Rate Transition/1 -> Kalmany/1(u)
  Rate Transition1/1 -> Kalmany/2(y)
  Rate Transition3/1 -> Kalmany/3(A)
  Rate Transition4/1 -> Kalmany/4(B)
  Rate Transition5/1 -> Kalmany/5(C)
  Rate Transition6/1 -> Kalmany/6(D)
  Kalmany/1(x) -> Rate Transition2/1
  Kalmany/2(K) -> Scope/1

== system main/Extended Kalman Filter/input linearization ==
  pose : Inport
  force : Inport  Port=2
  body 2 world 1 : MATLAB Function  TreatAsAtomicUnit=on
  force1 : Outport
  wires:
  pose/1 -> body 2 world 1/2(pose)
  body 2 world 1/1(pb) -> force1/1  "force"
  force/1 -> body 2 world 1/1(signal)

== system main/R2D2.1/traj generator ==
  pose : Inport
  Integrator : Integrator  InitialCondition=2
  trajectory gens : MATLAB Function  TreatAsAtomicUnit=on
  control point idx : Outport  PortDimensions=1
  previous control point : Outport  Port=2  PortDimensions=3
  next control point : Outport  Port=3  PortDimensions=3
  wires:
  trajectory gens/1(posei) -> previous control point/1
  pose/1 -> trajectory gens/1(fb)
  trajectory gens/3(added_idx) -> Integrator/1
  Integrator/1 -> control point idx/1, trajectory gens/2(idx)
  trajectory gens/2(posej) -> next control point/1

== system main/Repulsorlift Controller/gravitational force ==
  pose : Inport
  mass : Inport  Port=2
  Subsystem : Subsystem
      mask Display: image(imread("pictures/equations/gravitational_force.png"))
  gravitational force visualization : Scope  Commented=on
  "world 2 body " : MATLAB Function  TreatAsAtomicUnit=on
  gravitational force : Outport  PortDimensions=6
  wires:
  pose/1 -> "world 2 body "/2(pose), Subsystem/2(pose)  "pose"
  "world 2 body "/1(pb) -> gravitational force/1  "pose'"
  mass/1 -> Subsystem/1(mass)  "mass"
  Subsystem/2(Fg) -> "world 2 body "/1(signal)  "fg"
  Subsystem/1(z-axis gravitational force) -> gravitational force visualization/1  "fg_z"

== system main/Thrusters Controller/additional pitch PID ==
  u : Inport
  Gain1 : Gain  Gain=-1
  pitch PID1 : pid_lib/PID Controller  Controller=PID  Form=Parallel  TimeDomain=Continuous-time  UseExternalTs=off  SampleTime=-1  IntegratorMethod=Forward Euler  FilterMethod=Forward Euler  ControllerParametersSource=internal  P=1e-4  I=0  D=1e-3  UseFilter=on  N=100  TunerSelectOption=Transfer Function Based (PID Tuner App)  InitialConditionSource=internal  InitialConditionForIntegrator=0  InitialConditionForFilter=0  DifferentiatorICPrevScaledInput=0  ExternalReset=none  TrackingMode=off  Kt=1  LimitOutput=off  SatLimitsSource=internal  UpperSaturationLimit=inf  LowerSaturationLimit=-inf  LinearizeAsGain=on  AntiWindupMode=none  Kb=1  POutMin=[]  POutMax=[]  IOutMin=[]  IOutMax=[]  DOutMin=[]  DOutMax=[]  NOutMin=[]  NOutMax=[]  SumOutDataTypeStr=double  SumOutMin=[]  SumOutMax=[]  SaturationOutMin=[]  SaturationOutMax=[]  PParamMin=[]  PParamMax=[]  IParamMin=[]  IParamMax=[]  DParamMin=[]  DParamMax=[]  NParamMin=[]  NParamMax=[]  KbParamMin=[]  KbParamMax=[]  KtParamMin=[]  KtParamMax=[]  KbOutMin=[]  KbOutMax=[]  KtOutMin=[]  KtOutMax=[]  IntegratorOutMin=[]  IntegratorOutMax=[]  FilterOutMin=[]  FilterOutMax=[]  SumI1OutMin=[]  SumI1OutMax=[]  SumI2OutMin=[]  SumI2OutMax=[]  SumI3OutMin=[]  SumI3OutMax=[]  SumI4OutMin=[]  SumI4OutMax=[]  SumDOutMin=[]  SumDOutMax=[]  DifferentiatorOutMin=[]  DifferentiatorOutMax=[]  FilterDiffOutCoefMin=[]  FilterDiffOutCoefMax=[]  ReciprocalOutMin=[]  ReciprocalOutMax=[]  SumDenOutMin=[]  SumDenOutMax=[]  SumNumOutMin=[]  SumNumOutMax=[]  DivideOutMin=[]  DivideOutMax=[]  UdiffTsProdOutMin=[]  UdiffTsProdOutMax=[]  NTsProdOutMin=[]  NTsProdOutMax=[]  UintegralTsProdOutMin=[]  UintegralTsProdOutMax=[]  UngainTsProdOutMin=[]  UngainTsProdOutMax=[]  IntegratorContinuousStateAttributes=''  IntegratorStateMustResolveToSignalObject=off  IntegratorRTWStateStorageClass=Auto  FilterContinuousStateAttributes=''  FilterStateMustResolveToSignalObject=off  FilterRTWStateStorageClass=Auto  ParallelPVariant=InternalParameters  IdealPVariant=Disabled  IVariant=InternalParameters  DVariant=InternalParameters  IntegratorVariant=Continuous  SatVariant=Disabled  AWVariant=Passthrough  PCopyVariant=Disabled  TRVariant=Disabled  FdbkBlocksVariant=Forward  IdealPFdbkVariant=Disabled  SatFdbkVariant=Disabled  DerivativeFilterVariant=ContFilter  NVariant=InternalParameters  NCopyVariant=Disabled  FilterICVariant=InternalICsFilter  IntegratorICVariant=InternalICs  ExternalResetVariant=Disabled  TRSumVariant=Passthrough  SumFdbkVariant=Disabled  SumVariant=Sum_PID  TsampFilterVariant=InternalTs  TsampNgainVariant=Passthrough  TsampIntegralVariant=Passthrough  ExternalSaturationOutDataTypeStr=Inherit: Same as second input
  Out1 : Outport  PortDimensions=1
  wires:
  Gain1/1 -> Out1/1
  pitch PID1/1 -> Gain1/1
  u/1 -> pitch PID1/1

== system main/Thrusters Controller/compute additional pitch error ==
  velocity error (world-fixed frame) : Inport
  Abs : Abs
  Constant : Constant  Value=0
  Demux4 : Demux  Outputs=6
  Saturation : Saturate  UpperLimit=10  LowerLimit=-10
  Switch : Switch  Criteria=u2 > Threshold  Threshold=1
  addition pitch error : Outport  PortDimensions=1
  wires:
  Demux4/3 -> Abs/1, Switch/1
  Abs/1 -> Switch/2
  Constant/1 -> Switch/3
  Switch/1 -> Saturation/1
  Saturation/1 -> addition pitch error/1
  velocity error (world-fixed frame)/1 -> Demux4/1

== system main/Thrusters Controller/compute forward error ==
  velocity error : Inport
  Demux1 : Demux  Outputs=6
  forward error : Outport
  wires:
  Demux1/1 -> forward error/1
  velocity error/1 -> Demux1/1

== system main/Thrusters Controller/compute pitch error ==
  pose : Inport
  Constant2 : Constant  Value=0
  Demux5 : Demux  Outputs=6
  Sum1 : Sum  Inputs=|+-
  pitch error : Outport
  wires:
  Demux5/5 -> Sum1/2  "pitch"
  pose/1 -> Demux5/1
  Constant2/1 -> Sum1/1
  Sum1/1 -> pitch error/1  "pitch error"

== system main/Thrusters Controller/compute yaw error ==
  velocity_error : Inport
  pose : Inport  Port=2
  Abs : Abs
  Constant : Constant  Value=0
  Demux1 : Demux  Outputs=6
  Demux2 : Demux  Outputs=6
  Switch : Switch  Criteria=u2 > Threshold  Threshold=1
  vy : Outport
  wires:
  pose/1 -> Demux2/1
  Switch/1 -> vy/1
  Abs/1 -> Switch/2
  velocity_error/1 -> Demux1/1
  Demux1/1 -> Abs/1
  Constant/1 -> Switch/3
  Demux2/2 -> Switch/1  "vy"

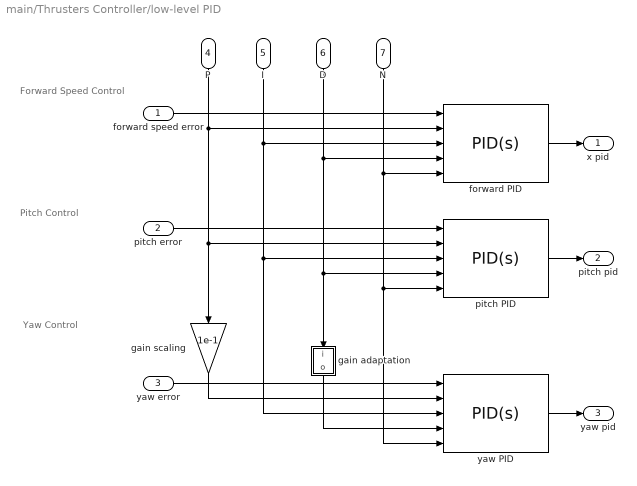
== system main/Thrusters Controller/low-level PID ==
  note: Yaw Control
  note: Pitch Control
  note: Forward Speed Control
  forward speed error : Inport
  pitch error : Inport  Port=2
  yaw error : Inport  Port=3
  P : Inport  Port=4
  I : Inport  Port=5
  D : Inport  Port=6
  N : Inport  Port=7
  forward PID : pid_lib/PID Controller  Controller=PID  Form=Parallel  TimeDomain=Continuous-time  UseExternalTs=off  SampleTime=-1  IntegratorMethod=Forward Euler  FilterMethod=Forward Euler  ControllerParametersSource=external  P=0.01  I=0  D=1  UseFilter=on  N=100  TunerSelectOption=Transfer Function Based (PID Tuner App)  InitialConditionSource=internal  InitialConditionForIntegrator=0  InitialConditionForFilter=0  DifferentiatorICPrevScaledInput=0  ExternalReset=none  TrackingMode=off  Kt=1  LimitOutput=off  SatLimitsSource=internal  UpperSaturationLimit=inf  LowerSaturationLimit=-inf  LinearizeAsGain=on  AntiWindupMode=none  Kb=1  POutMin=[]  POutMax=[]  IOutMin=[]  IOutMax=[]  DOutMin=[]  DOutMax=[]  NOutMin=[]  NOutMax=[]  SumOutMin=[]  SumOutMax=[]  SaturationOutMin=[]  SaturationOutMax=[]  PParamMin=[]  PParamMax=[]  IParamMin=[]  IParamMax=[]  DParamMin=[]  DParamMax=[]  NParamMin=[]  NParamMax=[]  KbParamMin=[]  KbParamMax=[]  KtParamMin=[]  KtParamMax=[]  KbOutMin=[]  KbOutMax=[]  KtOutMin=[]  KtOutMax=[]  IntegratorOutMin=[]  IntegratorOutMax=[]  FilterOutMin=[]  FilterOutMax=[]  SumI1OutMin=[]  SumI1OutMax=[]  SumI2OutMin=[]  SumI2OutMax=[]  SumI3OutMin=[]  SumI3OutMax=[]  SumI4OutMin=[]  SumI4OutMax=[]  SumDOutMin=[]  SumDOutMax=[]  DifferentiatorOutMin=[]  DifferentiatorOutMax=[]  FilterDiffOutCoefMin=[]  FilterDiffOutCoefMax=[]  ReciprocalOutMin=[]  ReciprocalOutMax=[]  SumDenOutMin=[]  SumDenOutMax=[]  SumNumOutMin=[]  SumNumOutMax=[]  DivideOutMin=[]  DivideOutMax=[]  UdiffTsProdOutMin=[]  UdiffTsProdOutMax=[]  NTsProdOutMin=[]  NTsProdOutMax=[]  UintegralTsProdOutMin=[]  UintegralTsProdOutMax=[]  UngainTsProdOutMin=[]  UngainTsProdOutMax=[]  IntegratorContinuousStateAttributes=''  IntegratorStateMustResolveToSignalObject=off  IntegratorRTWStateStorageClass=Auto  FilterContinuousStateAttributes=''  FilterStateMustResolveToSignalObject=off  FilterRTWStateStorageClass=Auto  ParallelPVariant=ExternalParameters  IdealPVariant=Disabled  IVariant=ExternalParameters  DVariant=ExternalParameters  IntegratorVariant=Continuous  SatVariant=Disabled  AWVariant=Passthrough  PCopyVariant=Disabled  TRVariant=Disabled  FdbkBlocksVariant=Forward  IdealPFdbkVariant=Disabled  SatFdbkVariant=Disabled  DerivativeFilterVariant=ContFilter  NVariant=ExternalParameters  NCopyVariant=Disabled  FilterICVariant=InternalICsFilter  IntegratorICVariant=InternalICs  ExternalResetVariant=Disabled  TRSumVariant=Passthrough  SumFdbkVariant=Disabled  SumVariant=Sum_PID  TsampFilterVariant=InternalTs  TsampNgainVariant=Passthrough  TsampIntegralVariant=Passthrough  ExternalSaturationOutDataTypeStr=Inherit: Same as second input
  gain adaptation : Subsystem
  gain scaling : Gain  Gain=1e-1
  pitch PID : pid_lib/PID Controller  Controller=PID  Form=Parallel  TimeDomain=Continuous-time  UseExternalTs=off  SampleTime=-1  IntegratorMethod=Forward Euler  FilterMethod=Forward Euler  ControllerParametersSource=external  P=0.01  I=0  D=1  UseFilter=on  N=100  TunerSelectOption=Transfer Function Based (PID Tuner App)  InitialConditionSource=internal  InitialConditionForIntegrator=0  InitialConditionForFilter=0  DifferentiatorICPrevScaledInput=0  ExternalReset=none  TrackingMode=off  Kt=1  LimitOutput=off  SatLimitsSource=internal  UpperSaturationLimit=inf  LowerSaturationLimit=-inf  LinearizeAsGain=on  AntiWindupMode=none  Kb=1  POutMin=[]  POutMax=[]  IOutMin=[]  IOutMax=[]  DOutMin=[]  DOutMax=[]  NOutMin=[]  NOutMax=[]  SumOutMin=[]  SumOutMax=[]  SaturationOutMin=[]  SaturationOutMax=[]  PParamMin=[]  PParamMax=[]  IParamMin=[]  IParamMax=[]  DParamMin=[]  DParamMax=[]  NParamMin=[]  NParamMax=[]  KbParamMin=[]  KbParamMax=[]  KtParamMin=[]  KtParamMax=[]  KbOutMin=[]  KbOutMax=[]  KtOutMin=[]  KtOutMax=[]  IntegratorOutMin=[]  IntegratorOutMax=[]  FilterOutMin=[]  FilterOutMax=[]  SumI1OutMin=[]  SumI1OutMax=[]  SumI2OutMin=[]  SumI2OutMax=[]  SumI3OutMin=[]  SumI3OutMax=[]  SumI4OutMin=[]  SumI4OutMax=[]  SumDOutMin=[]  SumDOutMax=[]  DifferentiatorOutMin=[]  DifferentiatorOutMax=[]  FilterDiffOutCoefMin=[]  FilterDiffOutCoefMax=[]  ReciprocalOutMin=[]  ReciprocalOutMax=[]  SumDenOutMin=[]  SumDenOutMax=[]  SumNumOutMin=[]  SumNumOutMax=[]  DivideOutMin=[]  DivideOutMax=[]  UdiffTsProdOutMin=[]  UdiffTsProdOutMax=[]  NTsProdOutMin=[]  NTsProdOutMax=[]  UintegralTsProdOutMin=[]  UintegralTsProdOutMax=[]  UngainTsProdOutMin=[]  UngainTsProdOutMax=[]  IntegratorContinuousStateAttributes=''  IntegratorStateMustResolveToSignalObject=off  IntegratorRTWStateStorageClass=Auto  FilterContinuousStateAttributes=''  FilterStateMustResolveToSignalObject=off  FilterRTWStateStorageClass=Auto  ParallelPVariant=ExternalParameters  IdealPVariant=Disabled  IVariant=ExternalParameters  DVariant=ExternalParameters  IntegratorVariant=Continuous  SatVariant=Disabled  AWVariant=Passthrough  PCopyVariant=Disabled  TRVariant=Disabled  FdbkBlocksVariant=Forward  IdealPFdbkVariant=Disabled  SatFdbkVariant=Disabled  DerivativeFilterVariant=ContFilter  NVariant=ExternalParameters  NCopyVariant=Disabled  FilterICVariant=InternalICsFilter  IntegratorICVariant=InternalICs  ExternalResetVariant=Disabled  TRSumVariant=Passthrough  SumFdbkVariant=Disabled  SumVariant=Sum_PID  TsampFilterVariant=InternalTs  TsampNgainVariant=Passthrough  TsampIntegralVariant=Passthrough  ExternalSaturationOutDataTypeStr=Inherit: Same as second input
  yaw PID : pid_lib/PID Controller  Controller=PID  Form=Parallel  TimeDomain=Continuous-time  UseExternalTs=off  SampleTime=-1  IntegratorMethod=Forward Euler  FilterMethod=Forward Euler  ControllerParametersSource=external  P=0.01  I=0  D=1  UseFilter=on  N=100  TunerSelectOption=Transfer Function Based (PID Tuner App)  InitialConditionSource=internal  InitialConditionForIntegrator=0  InitialConditionForFilter=0  DifferentiatorICPrevScaledInput=0  ExternalReset=none  TrackingMode=off  Kt=1  LimitOutput=off  SatLimitsSource=internal  UpperSaturationLimit=inf  LowerSaturationLimit=-inf  LinearizeAsGain=on  AntiWindupMode=none  Kb=1  POutMin=[]  POutMax=[]  IOutMin=[]  IOutMax=[]  DOutMin=[]  DOutMax=[]  NOutMin=[]  NOutMax=[]  SumOutMin=[]  SumOutMax=[]  SaturationOutMin=[]  SaturationOutMax=[]  PParamMin=[]  PParamMax=[]  IParamMin=[]  IParamMax=[]  DParamMin=[]  DParamMax=[]  NParamMin=[]  NParamMax=[]  KbParamMin=[]  KbParamMax=[]  KtParamMin=[]  KtParamMax=[]  KbOutMin=[]  KbOutMax=[]  KtOutMin=[]  KtOutMax=[]  IntegratorOutMin=[]  IntegratorOutMax=[]  FilterOutMin=[]  FilterOutMax=[]  SumI1OutMin=[]  SumI1OutMax=[]  SumI2OutMin=[]  SumI2OutMax=[]  SumI3OutMin=[]  SumI3OutMax=[]  SumI4OutMin=[]  SumI4OutMax=[]  SumDOutMin=[]  SumDOutMax=[]  DifferentiatorOutMin=[]  DifferentiatorOutMax=[]  FilterDiffOutCoefMin=[]  FilterDiffOutCoefMax=[]  ReciprocalOutMin=[]  ReciprocalOutMax=[]  SumDenOutMin=[]  SumDenOutMax=[]  SumNumOutMin=[]  SumNumOutMax=[]  DivideOutMin=[]  DivideOutMax=[]  UdiffTsProdOutMin=[]  UdiffTsProdOutMax=[]  NTsProdOutMin=[]  NTsProdOutMax=[]  UintegralTsProdOutMin=[]  UintegralTsProdOutMax=[]  UngainTsProdOutMin=[]  UngainTsProdOutMax=[]  IntegratorContinuousStateAttributes=''  IntegratorStateMustResolveToSignalObject=off  IntegratorRTWStateStorageClass=Auto  FilterContinuousStateAttributes=''  FilterStateMustResolveToSignalObject=off  FilterRTWStateStorageClass=Auto  ParallelPVariant=ExternalParameters  IdealPVariant=Disabled  IVariant=ExternalParameters  DVariant=ExternalParameters  IntegratorVariant=Continuous  SatVariant=Disabled  AWVariant=Passthrough  PCopyVariant=Disabled  TRVariant=Disabled  FdbkBlocksVariant=Forward  IdealPFdbkVariant=Disabled  SatFdbkVariant=Disabled  DerivativeFilterVariant=ContFilter  NVariant=ExternalParameters  NCopyVariant=Disabled  FilterICVariant=InternalICsFilter  IntegratorICVariant=InternalICs  ExternalResetVariant=Disabled  TRSumVariant=Passthrough  SumFdbkVariant=Disabled  SumVariant=Sum_PID  TsampFilterVariant=InternalTs  TsampNgainVariant=Passthrough  TsampIntegralVariant=Passthrough  ExternalSaturationOutDataTypeStr=Inherit: Same as second input
  x pid : Outport  Unit=1
  pitch pid : Outport  Port=2  Unit=1
  yaw pid : Outport  Port=3  Unit=1
  wires:
  P/1 -> forward PID/2, gain scaling/1, pitch PID/2
  N/1 -> yaw PID/5, pitch PID/5, forward PID/5
  I/1 -> forward PID/3, pitch PID/3, yaw PID/3
  D/1 -> pitch PID/4, gain adaptation/1(i), forward PID/4
  pitch error/1 -> pitch PID/1
  forward speed error/1 -> forward PID/1
  gain scaling/1 -> yaw PID/2
  pitch PID/1 -> pitch pid/1
  yaw PID/1 -> yaw pid/1
  yaw error/1 -> yaw PID/1
  gain adaptation/1(o) -> yaw PID/4
  forward PID/1 -> x pid/1
